simulink subsystem "combiner"  (R2021b)
settings: Solver=VariableStepAuto  StartTime=0.0  StopTime=10.0  RelTol=1e-3
undefined symbols (not defined in the file or in its folder): antenna_num, stream_num
settings Model: Creator=torha  LastModifiedBy=torha

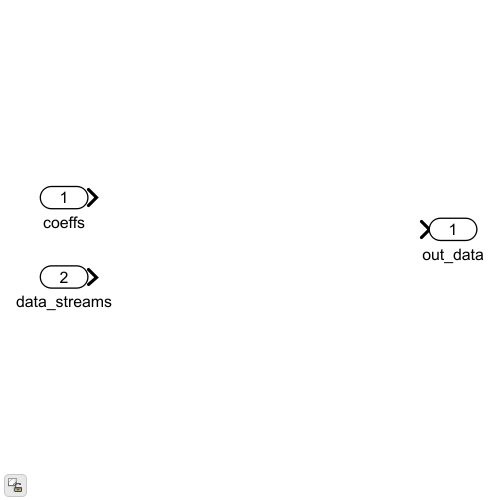
[thumbnail: Simulink's stored preview of the top-level diagram]
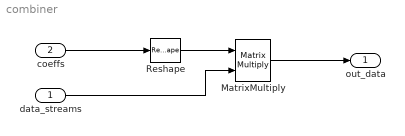
== system combiner ==
  data_streams : Inport
  coeffs : Inport  Port=2
  MatrixMultiply : Product  Multiplication=Matrix(*)
  Reshape : Reshape  OutputDimensionality=Customize  OutputDimensions=[stream_num, antenna_num]
  out_data : Outport
  wires:
  data_streams/1 -> MatrixMultiply/2
  MatrixMultiply/1 -> out_data/1
  Reshape/1 -> MatrixMultiply/1
  coeffs/1 -> Reshape/1
